simulink model "fcs_lab_05_model_01"  (R2014b)
settings: Solver=ode45  StartTime=0.0  StopTime=10.0  RelTol=1e-3
values from neighbouring files (symbols this model uses):
  B1 = 20    [fcs_lab_05_model_01_test.m]
  B2 = 30    [fcs_lab_05_model_01_test.m]
  B3 = 30    [fcs_lab_05_model_01_test.m]
  F = 300    [fcs_lab_05_model_01_test.m]
  K1 = 15    [fcs_lab_05_model_01_test.m]
  K2 = 15    [fcs_lab_05_model_01_test.m]
  M1 = 750    [fcs_lab_05_model_01_test.m]
  M2 = 750    [fcs_lab_05_model_01_test.m]
settings Model: Creator=Mashkoor Ahmed  LastModifiedBy=Mashkoor Ahmed

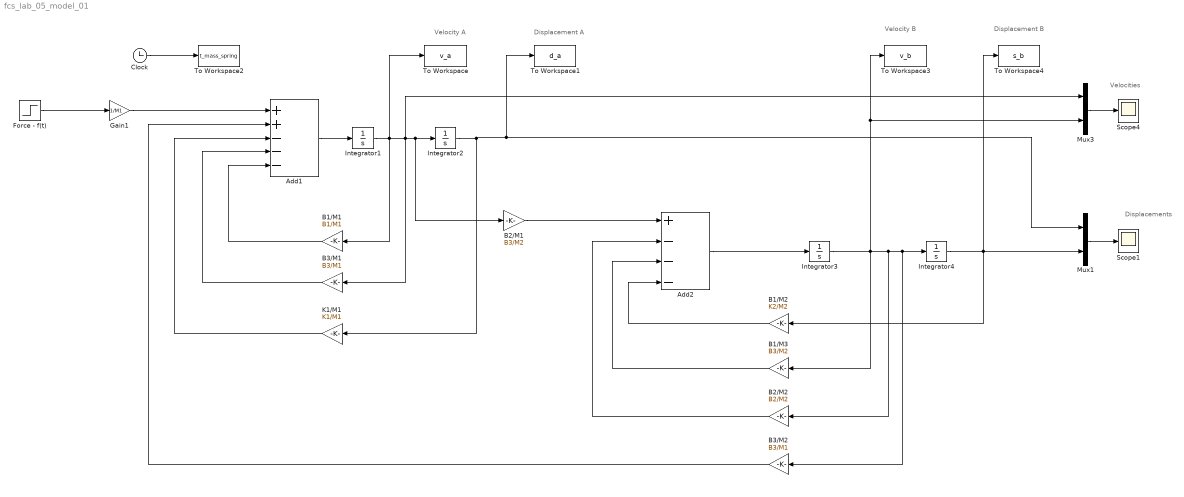
== system fcs_lab_05_model_01 ==
  note: Displacement B
  note: Velocity B
  note: Velocities
  note: Displacements
  note: Displacement A
  note: Velocity A
  Add1 : Sum  Inputs=++---
  Add2 : Sum  Inputs=+---
  B1/M1 : Gain  Gain=B1/M1
  B1/M2 : Gain  Gain=K2/M2
  B1/M3 : Gain  Gain=B3/M2
  B2/M1 : Gain  Gain=B3/M2
  B2/M2 : Gain  Gain=B2/M2
  B3/M1 : Gain  Gain=B3/M1
  B3/M2 : Gain  Gain=B3/M1
  Clock : Clock
  Force - f(t) : Step  After=F  SampleTime=0
  Gain1 : Gain  Gain=1/M1
  Integrator{1..4} (4 alike) : Integrator
  K1/M1 : Gain  Gain=K1/M1
  Mux1 : Mux  Inputs=2
  Mux3 : Mux  Inputs=2
  Scope1 : Scope
      settings: YMin=-5.00203  YMax=33.83101
  Scope4 : Scope
      settings: YMin=-1.56348  YMax=2.49523
  To Workspace : ToWorkspace  VariableName=v_a  SaveFormat=Timeseries  SampleTime=-1
  To Workspace1 : ToWorkspace  VariableName=d_a  SaveFormat=Timeseries  SampleTime=-1
  To Workspace2 : ToWorkspace  VariableName=t_mass_spring  SaveFormat=Timeseries  SampleTime=-1
  To Workspace3 : ToWorkspace  VariableName=v_b  SaveFormat=Timeseries  SampleTime=-1
  To Workspace4 : ToWorkspace  VariableName=s_b  SaveFormat=Timeseries  SampleTime=-1
  wires:
  Add1/1 -> Integrator1/1
  Integrator1/1 -> B1/M1/1, Mux3/1, B3/M1/1, B2/M1/1, Integrator2/1, To Workspace/1
  Mux3/1 -> Scope4/1
  Integrator2/1 -> Mux1/1, To Workspace1/1, K1/M1/1
  B1/M1/1 -> Add1/5
  K1/M1/1 -> Add1/3
  Gain1/1 -> Add1/1
  Force - f(t)/1 -> Gain1/1
  Clock/1 -> To Workspace2/1
  B3/M1/1 -> Add1/4
  Add2/1 -> Integrator3/1
  Integrator4/1 -> To Workspace4/1, Mux1/2, B1/M2/1
  B3/M2/1 -> Add1/2
  B1/M2/1 -> Add2/4
  B1/M3/1 -> Add2/3
  B2/M2/1 -> Add2/2
  Integrator3/1 -> To Workspace3/1, Mux3/2, B1/M3/1, B3/M2/1, Integrator4/1, B2/M2/1
  Mux1/1 -> Scope1/1
  B2/M1/1 -> Add2/1
